simulink model "Supply_Chain_III"  (R2018b)
settings: Solver=VariableStepAuto  StartTime=0.0  StopTime=n_T  RelTol=1e-3
undefined symbols (not defined in the file or in its folder): m, MTBF_h, n, yoi
libraries: simulink x6
settings Model: Creator=Jorrit de Jong  LastModifiedBy=Jorrit de Jong

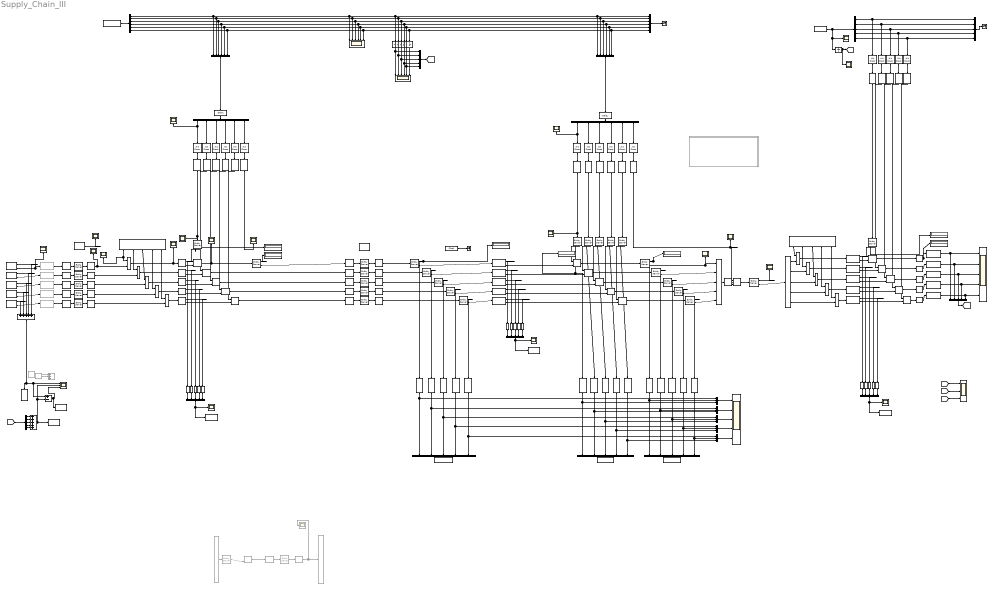
== system Supply_Chain_III ==
  note: KPI to indicate the in-time or delayed deliveries
  note: KPI to indicate the component availability on AI
  note: Performance measurement
  note: Local Warehouse
  note: Scopes
  note: KPI to indicate demanded terminal capacity
  note: Shedule Agent
  note: Control agent
  note: Terminal
  note: Island
  note: Performance measurement JIT
  note: Performance measurement
  note: Control agent
  note: Nr of parts departed
  note: Failure Agent
  note: Performance measurement
  note: KPI to measure the inventory level relative to the sigma level
  note: Source
  Add : Sum  Inputs=+++++
  Add1 : Sum  Inputs=+++++
  Add2 : Sum  Inputs=+-
  Add3 : Sum  Commented=on  Inputs=+++
  Arrived spares : Display
  Blade terminator : EntityTerminator  InputPortMessageModes=m  NumberEntitiesArrived=on
      settings: OutputPortMap=o0
  C terminator : EntityTerminator  InputPortMessageModes=m  NumberEntitiesArrived=on
      settings: OutputPortMap=o0
  Components arrived : Scope  NumInputPorts=5
  Constant : Constant  Commented=on  Value=5*20
  Constant1 : Constant  Commented=on  Value=5*20
  Counter : EntityServer  InputPortMessageModes=m  OutputPortMessageModes=n,m  Capacity=inf  ServiceTimeValue=0  NumberEntitiesDeparted=on
      settings: OutputPortMap=o0,o9
  Counter2 : EntityServer  InputPortMessageModes=m  OutputPortMessageModes=n,m  Capacity=inf  ServiceTimeValue=0  NumberEntitiesDeparted=on
      settings: OutputPortMap=o0,o9
  D terminator : EntityTerminator  InputPortMessageModes=m  NumberEntitiesArrived=on
      settings: OutputPortMap=o0
  DC transport signal : Scope
  DC trigger : Scope
  Data Type Conversion{,1..34} (35 alike) : DataTypeConversion
  Demand - delivery flow : Scope  NumInputPorts=3
  Demux : Demux  Outputs=6
  Demux1 : Demux  Outputs=5
  Demux2 : Demux  Outputs=5
  Demux3 : Demux  Outputs=6
  Demux5 : Demux  Outputs=6
  Departed/Arrived components : Scope  NumInputPorts=3
  Digital Clock : DigitalClock
  Display : Display
  Display1 : Display
  Display2 : Display
  E terminator : EntityTerminator  InputPortMessageModes=m  NumberEntitiesArrived=on
      settings: OutputPortMap=o0
  Entity Input Switch : EntityInputSwitch  Commented=on  InputPortMessageModes=m,m,m,m,m  OutputPortMessageModes=m  NumberInputPorts=5
      settings: InputPortMap=u1,u2,u3,u4,u5
  Entity Input Switch{1..5,7..11} (10 alike) : EntityInputSwitch  InputPortMessageModes=m,m  OutputPortMessageModes=m
  Entity Input Switch6 : EntityInputSwitch  InputPortMessageModes=m,m,m,m,m  OutputPortMessageModes=m  NumberInputPorts=5
      settings: InputPortMap=u1,u2,u3,u4,u5
  Entity Output Switch : EntityOutputSwitch  InputPortMessageModes=m  OutputPortMessageModes=m,m,m,m,m  NumberOutputPorts=5  SwitchingCriterion=From attribute  SwitchAttributeName=PartNumber
      settings: OutputPortMap=o0,o1,o2,o3,o4
  Entity Output Switch1 : EntityOutputSwitch  Commented=on  InputPortMessageModes=m  OutputPortMessageModes=m,m,m,m,m  NumberOutputPorts=5  SwitchingCriterion=From attribute  SwitchAttributeName=PartNumber
      settings: OutputPortMap=o0,o1,o2,o3,o4
  Entity Gate{,1..9,11..16} (16 alike) : EntityGate  InputPortMessageModes=m,m  OutputPortMessageModes=m  OperatingMode=Release gate
  Entity Gate10 : EntityGate  Commented=on  InputPortMessageModes=m,m  OutputPortMessageModes=m  OperatingMode=Release gate
  Entity Generator : EntityGenerator  OutputPortMessageModes=n,m  Period=MTBF_h(1,yoi)  AttributeName=PartNumber  NumberEntitiesDeparted=on  EntityType=Structured  EntityTypeName=Part
      settings: OutputPortMap=o0,o3
  Entity Generator1 : EntityGenerator  OutputPortMessageModes=n,m  Period=MTBF_h(2,yoi)  AttributeName=PartNumber  AttributeInitialValue=2  NumberEntitiesDeparted=on  EntityType=Structured  EntityTypeName=Part
      settings: OutputPortMap=o0,o3
  Entity Generator{5..16,18..22} (17 alike) : EntityGenerator  InputPortMessageModes=m  OutputPortMessageModes=m  GenerationMethod=Event-based  AttributeName=entity  AttributeInitialValue=0  EntityTypeName=Entity
      settings: InputPortMap=u0
  Entity Generator2 : EntityGenerator  OutputPortMessageModes=n,m  Period=MTBF_h(3,yoi)  AttributeName=PartNumber  AttributeInitialValue=3  NumberEntitiesDeparted=on  EntityType=Structured  EntityTypeName=Part
      settings: OutputPortMap=o0,o3
  Entity Generator3 : EntityGenerator  OutputPortMessageModes=n,m  Period=MTBF_h(4,yoi)  AttributeName=PartNumber  AttributeInitialValue=4  NumberEntitiesDeparted=on  EntityType=Structured  EntityTypeName=Part
      settings: OutputPortMap=o0,o3
  Entity Generator4 : EntityGenerator  OutputPortMessageModes=n,m  Period=MTBF_h(5,yoi)  AttributeName=PartNumber  AttributeInitialValue=5  NumberEntitiesDeparted=on  EntityType=Structured  EntityTypeName=Part
      settings: OutputPortMap=o0,o3
  Entity Queue{,1..9} (10 alike) : EntityQueue  InputPortMessageModes=m  OutputPortMessageModes=n,m  Capacity=20  NumberEntitiesInBlock=on
      settings: OutputPortMap=o1,o5
  Entity Queue{10..14} (5 alike) : EntityQueue  Commented=through  InputPortMessageModes=m  OutputPortMessageModes=m  Capacity=1
      settings: OutputPortMap=o5
  Entity Server{,1..3,9..20} (16 alike) : EntityServer  InputPortMessageModes=m  OutputPortMessageModes=n,m  Capacity=inf  ServiceTimeValue=0  NumberEntitiesDeparted=on
      settings: OutputPortMap=o0,o9
  Entity Server{4..8} (5 alike) : EntityServer  InputPortMessageModes=m  OutputPortMessageModes=m  Capacity=inf  ServiceTimeSource=MATLAB action  ServiceTimeValue=20  ServiceTimeAction=dt = normrnd(D(1,3),ts_sigma_distance(1,3));
  Entity Store{,1..4} (5 alike) : EntityStore  InputPortMessageModes=m  OutputPortMessageModes=n,m  Capacity=20  NumberEntitiesInBlock=on
      settings: OutputPortMap=o1,o4
  Entity Store6 : EntityStore  InputPortMessageModes=m  OutputPortMessageModes=m  Capacity=inf
      settings: OutputPortMap=o4
  Failures : Display
  Failures cumulated : Scope
  Failures3 : Display
  From Workspace : FromWorkspace  VariableName=Failure_events  SampleTime=0
  From Workspace1 : FromWorkspace  VariableName=Schedule_data  SampleTime=0
  Gearbox terminator : EntityTerminator  InputPortMessageModes=m  NumberEntitiesArrived=on
      settings: OutputPortMap=o0
  Hit Crossing{,1..16} (17 alike) : HitCross  OutputPortMessageModes=m  HitCrossingDirection=rising  HitCrossingOutputType=Message
  Ini supply creator : Subsystem
  Ini supply creator1 : Subsystem
  Integrator{,3..8} (7 alike) : Integrator
  Inventory level island : Scope
  Inventory level local warehouse : Scope
  Inventory level terminal : Scope
  JIT Scope : Scope  NumInputPorts=5
  Loading : EntityServer  Commented=on  InputPortMessageModes=m  OutputPortMessageModes=m  Capacity=inf  ServiceTimeValue=1
  Mux : Mux  Inputs=6
  Mux{1,4..9,15,17} (9 alike) : Mux  Inputs=5
  Mux10 : Mux  Inputs=6
  Mux{3,11..14} (5 alike) : Mux  Inputs=3
  Mux2 : Mux  Inputs=6
  Overall DC releaser : Scope
  Passed components : Display
  Post DC trigger : Scope
  Pre DC storage{,1..4} (5 alike) : Scope
  Resource Acquirer{,1..4} (5 alike) : EntityResourceAcquirer  InputPortMessageModes=m  OutputPortMessageModes=m  ResourceName=LD_trucks
      settings: OutputPortMap=o3
  Resource Acquirer{6..10} (5 alike) : EntityResourceAcquirer  InputPortMessageModes=m  OutputPortMessageModes=m
      settings: OutputPortMap=o3
  Resource Acquirer5 : EntityResourceAcquirer  Commented=on  InputPortMessageModes=m  OutputPortMessageModes=m
      settings: OutputPortMap=o3
  Resource Releaser{,1..4} (5 alike) : EntityResourceReleaser  InputPortMessageModes=m  OutputPortMessageModes=m  ResourceToRelease=Selected  ResourceName=LD_trucks
  Resource Releaser{6..10} (5 alike) : EntityResourceReleaser  InputPortMessageModes=m  OutputPortMessageModes=m
  Resource Releaser5 : EntityResourceReleaser  Commented=on  InputPortMessageModes=m  OutputPortMessageModes=m
  Resource Pool : EntityResourcePool  ResourceName=LD_trucks  ResourceAmount=30  AverageUtilization=on
      settings: OutputPortMap=o1
  Resource Pool1 : EntityResourcePool  ResourceAmount=n_R
  Road transport : EntityServer  Commented=on  InputPortMessageModes=m  OutputPortMessageModes=m  Capacity=inf  ServiceTimeSource=MATLAB action  ServiceTimeValue=20  ServiceTimeAction=dt = normrnd(D(3,4),ts_sigma_distance(3,4));
  Road transport troughput : Scope  Commented=on
  Road transport{1..5} (5 alike) : EntityServer  InputPortMessageModes=m  OutputPortMessageModes=m  Capacity=inf  ServiceTimeSource=MATLAB action  ServiceTimeValue=20  ServiceTimeAction=dt = normrnd(D(3,4),ts_sigma_distance(3,4));
  Schedule data : Scope  NumInputPorts=6
  Schedule data accumulated : Scope  NumInputPorts=6
  Scope4 : Scope
  Sea Transport : EntityServer  InputPortMessageModes=m  OutputPortMessageModes=n,m  Capacity=inf  ServiceTimeSource=MATLAB action  ServiceTimeValue=50  ServiceTimeAction=dt = normrnd(ts_vessel,2);  NumberEntitiesDeparted=on
      settings: OutputPortMap=o0,o9
  Sea transport post releaser : Scope
  Sea transport releaser : Scope
  Sea transport signal : Scope
  Sea transport sope : Scope
  Sea transport trigger : Scope
  Switched transport delay for linearization : TransportDelay  DelayTime=3  PadeOrder=1
  Switched transport delay for linearization1 : TransportDelay  PadeOrder=1
  Terminal trigger system : Subsystem  Commented=on
  Terminator1 : Terminator
  Terminator2 : Terminator
  Terminator4 : Terminator
  To Workspace : ToWorkspace  VariableName=inventory_level_island
      settings: Save2DSignal=2-D array (concatenate along first dimension)
  To Workspace1 : ToWorkspace  VariableName=com_caller
      settings: Save2DSignal=2-D array (concatenate along first dimension)
  To Workspace2 : ToWorkspace  VariableName=com_released
      settings: Save2DSignal=2-D array (concatenate along first dimension)
  To Workspace3 : ToWorkspace  VariableName=com_arrivals
      settings: Save2DSignal=2-D array (concatenate along first dimension)
  To Workspace4 : ToWorkspace  VariableName=inventory_level_terminal
      settings: Save2DSignal=2-D array (concatenate along first dimension)
  To Workspace5 : ToWorkspace  VariableName=inventory_level_LW
      settings: Save2DSignal=2-D array (concatenate along first dimension)
  To Workspace6 : ToWorkspace  VariableName=departed_comps
      settings: Save2DSignal=2-D array (concatenate along first dimension)
  To Workspace7 : ToWorkspace  VariableName=arrived_comps
      settings: Save2DSignal=2-D array (concatenate along first dimension)
  To Workspace8 : ToWorkspace  VariableName=n_comps_in_sc
      settings: Save2DSignal=2-D array (concatenate along first dimension)
  wires:
  Data Type Conversion15/1 -> Mux6/5  "Transformers"
  Entity Queue6/1 -> Data Type Conversion9/1
  Counter/1 -> Passed components/1
  Hit Crossing7/1 -> Entity Generator12/1
  Entity Queue2/2 -> Entity Gate2/2
  Entity Queue1/2 -> Entity Gate1/2
  Entity Gate1/1 -> Gearbox terminator/1
  Entity Gate/1 -> Blade terminator/1
  Hit Crossing1/1 -> Entity Generator6/1
  Demux/1 -> Schedule data/1, Integrator3/1, Mux2/1, Mux/1, Mux10/1  "A"
  Entity Output Switch/5 -> Entity Input Switch5/2
  Resource Releaser/1 -> Entity Input Switch7/2, Pre DC storage4/1
  Entity Generator2/1 -> Add/3
  Entity Input Switch3/1 -> Entity Queue2/1
  Constant/1 -> Add3/1
  Entity Store3/1 -> Data Type Conversion14/1
  Constant1/1 -> Add3/2
  Demux2/1 -> Add1/1
  Integrator3/1 -> Mux17/1, Schedule data accumulated/1
  Entity Server5/1 -> Resource Releaser1/1
  Demux2/2 -> Add1/2
  Entity Queue8/1 -> Data Type Conversion11/1
  Entity Server3/1 -> Display2/1, Data Type Conversion2/1
  Data Type Conversion32/1 -> Mux15/3, Components arrived/3
  Entity Server/1 -> Display/1, Data Type Conversion1/1
  Integrator4/1 -> Mux17/2, Schedule data accumulated/2
  Entity Gate7/1 -> Resource Acquirer8/1
  Entity Server11/2 -> Entity Queue8/1
  Hit Crossing4/1 -> Entity Generator9/1
  Data Type Conversion31/1 -> Mux15/2, Components arrived/2
  Data Type Conversion4/1 -> Mux4/2  "Gearboxes"
  Entity Generator14/1 -> Entity Gate8/1
  Demux2/3 -> Add1/3
  Entity Queue4/2 -> Entity Gate4/2
  Entity Generator3/1 -> Add/2
  Add/1 -> To Workspace6/1, Add2/1, Departed/Arrived components/1  "Departs"
  Integrator8/1 -> Schedule data accumulated/6
  Demux/2 -> Schedule data/2, Integrator4/1, Mux2/2, Mux/2, Mux10/2  "B"
  [Sche_comps] -> Demand - delivery flow/2  "Scheduled"
  Entity Generator1/1 -> Add/4
  Entity Server6/1 -> Resource Releaser2/1
  Resource Releaser1/1 -> Entity Input Switch8/2
  Entity Gate9/1 -> Resource Acquirer10/1
  Entity Queue3/1 -> Data Type Conversion6/1
  Data Type Conversion34/1 -> Mux15/5, Components arrived/5
  Demux3/3 -> Hit Crossing8/1
  Demux3/5 -> Hit Crossing10/1
  Entity Queue10/1 -> Resource Acquirer/1
  Resource Acquirer3/1 -> Entity Server7/1
  Mux11/1 -> JIT Scope/2  "Gearboxes"
  Entity Queue7/1 -> Data Type Conversion10/1
  Resource Acquirer1/1 -> Entity Server5/1
  Entity Queue11/1 -> Resource Acquirer1/1
  Entity Queue12/1 -> Resource Acquirer2/1
  Mux15/1 -> [Arr_comps]
  Entity Server1/1 -> Failures/1
  Data Type Conversion12/1 -> Mux5/5  "Transformers"
  Entity Server12/2 -> Entity Queue9/1
  Data Type Conversion16/1 -> Mux6/1  "Blades"
  Resource Acquirer2/1 -> Entity Server6/1
  Entity Queue8/2 -> Entity Gate14/2
  Data Type Conversion33/1 -> Mux15/4, Components arrived/4
  Entity Generator13/1 -> Entity Gate7/1
  Integrator7/1 -> Mux17/5, Schedule data accumulated/5
  Data Type Conversion3/1 -> Mux4/1  "Blades"
  Gearbox terminator/1 -> Data Type Conversion31/1
  Entity Gate3/1 -> D terminator/1
  Data Type Conversion30/1 -> Mux15/1, Components arrived/1
  Data Type Conversion5/1 -> Mux4/3  "Generators"
  Road transport1/1 -> Resource Releaser6/1
  Entity Queue3/2 -> Entity Gate3/2
  Entity Server15/1 -> Data Type Conversion24/1
  Integrator/1 -> Failures cumulated/1, [Fail_comps]
  Data Type Conversion7/1 -> Mux4/5  "Transformers"
  Entity Generator22/1 -> Entity Gate4/1
  Integrator5/1 -> Mux17/3, Schedule data accumulated/3
  D terminator/1 -> Data Type Conversion33/1
  Entity Generator19/1 -> Entity Gate1/1
  Data Type Conversion20/1 -> Mux13/1, Mux9/4  "Arrivals"
  Hit Crossing/1 -> Entity Generator5/1
  Demux/6 -> Schedule data/6, Integrator8/1, Mux2/6, Mux/6, Mux10/6  "t"
  From Workspace/1 -> Integrator/1, Scope4/1, Demux1/1
  Entity Gate2/1 -> C terminator/1
  Resource Releaser4/1 -> Entity Input Switch11/2
  Demux/3 -> Schedule data/3, Integrator5/1, Mux2/3, Mux/3, Mux10/3  "C"
  Demux2/4 -> Add1/4
  Hit Crossing14/1 -> Entity Generator20/1
  Demux3/6 -> Hit Crossing11/1
  Mux3/1 -> JIT Scope/1  "Blades"
  Resource Acquirer/1 -> Entity Server4/1
  E terminator/1 -> Data Type Conversion34/1
  Resource Releaser2/1 -> Entity Input Switch9/2
  Entity Generator21/1 -> Entity Gate3/1
  Demux5/1 -> Hit Crossing/1, Sea transport signal/1
  Mux/1 -> Terminator4/1
  Demux/4 -> Schedule data/4, Integrator6/1, Mux2/4, Mux/4, Mux10/4  "D"
  Resource Releaser3/1 -> Entity Input Switch10/2
  Digital Clock/1 -> Terminator1/1
  Counter/2 -> Resource Acquirer6/1
  Data Type Conversion11/1 -> Mux5/4  "Rotorhubs"
  Ini supply creator1/3(C) -> Entity Input Switch9/1
  Mux2/1 -> Switched transport delay for linearization/1
  Entity Generator15/1 -> Entity Gate9/1
  Entity Queue9/1 -> Data Type Conversion12/1
  Entity Gate5/1 -> Post DC trigger/1, Counter/1
  Entity Generator10/1 -> Entity Gate16/1, Sea transport releaser/1
  Mux10/1 -> Switched transport delay for linearization1/1
  Hit Crossing16/1 -> Entity Generator22/1
  From Workspace1/1 -> Demux/1
  Entity Generator16/1 -> Overall DC releaser/1
  Hit Crossing15/1 -> Entity Generator21/1
  Demux3/2 -> Hit Crossing7/1
  Demux1/2 -> Mux1/2, Hit Crossing13/1  "B"
  Hit Crossing10/1 -> Entity Generator15/1
  Demux1/1 -> Mux1/1, Hit Crossing12/1  "A"
  Mux5/1 -> To Workspace4/1, Inventory level terminal/1
  Mux17/1 -> [Sche_comps]
  Entity Generator11/1 -> DC trigger/1, Counter2/1
  Entity Output Switch/3 -> Entity Input Switch3/2
  Entity Input Switch11/1 -> Entity Store4/1
  Entity Generator4/2 -> Entity Queue14/1
  Data Type Conversion8/1 -> Mux5/1  "Blades"
  Mux9/1 -> To Workspace3/1
  Entity Generator7/1 -> Entity Server18/1
  Entity Output Switch/2 -> Entity Input Switch2/2
  Demux1/4 -> Mux1/4, Hit Crossing15/1  "D"
  Entity Generator8/1 -> Entity Server19/1
  Entity Generator5/1 -> Sea transport trigger/1, Entity Server2/1
  Blade terminator/1 -> Arrived spares/1, Data Type Conversion30/1
  Hit Crossing9/1 -> Entity Generator14/1
  Demux1/5 -> Mux1/5, Hit Crossing16/1  "E"
  Data Type Conversion23/1 -> Mux8/3, Mux12/2  "Released"
  Switched transport delay for linearization1/1 -> Demux3/1
  Entity Server10/2 -> Entity Queue7/1
  Switched transport delay for linearization/1 -> Demux5/1
  Data Type Conversion21/1 -> Mux9/5, Mux14/1  "Arrivals"
  Hit Crossing12/1 -> Entity Generator18/1
  [Fail_comps] -> Demand - delivery flow/1  "Failures"
  Add2/1 -> To Workspace8/1, Departed/Arrived components/3  "Result"
  Entity Server/2 -> Entity Input Switch6/1, Sea transport post releaser/1
  Demux1/3 -> Mux1/3, Hit Crossing14/1  "C"
  C terminator/1 -> Data Type Conversion32/1
  Data Type Conversion10/1 -> Mux5/3  "Generators"
  Demux3/1 -> Hit Crossing6/1, DC transport signal/1
  Entity Store/2 -> Entity Gate5/2
  Entity Queue14/1 -> Resource Acquirer4/1
  Data Type Conversion1/1 -> Mux3/2, Mux8/1  "Released"
  Entity Server1/2 -> Entity Gate/1
  Mux12/1 -> JIT Scope/3  "Generators"
  Data Type Conversion18/1 -> Mux11/1, Mux9/2  "Arrivals"
  Entity Server14/1 -> Data Type Conversion23/1
  Entity Queue4/1 -> Data Type Conversion7/1
  Entity Generator/2 -> Pre DC storage2/1, Entity Queue10/1
  Entity Store4/1 -> Data Type Conversion15/1
  Entity Gate4/1 -> E terminator/1
  Hit Crossing8/1 -> Entity Generator13/1
  Entity Server4/1 -> Resource Releaser/1
  Demux5/5 -> Hit Crossing4/1
  Entity Server13/1 -> Data Type Conversion22/1
  Data Type Conversion25/1 -> Mux8/5, Mux14/2  "Released"
  Entity Generator1/2 -> Entity Queue11/1
  Entity Queue5/1 -> Data Type Conversion8/1
  Mux6/1 -> To Workspace5/1, Inventory level local warehouse/1
  Data Type Conversion22/1 -> Mux11/2, Mux8/2  "Released"
  Mux14/1 -> JIT Scope/5  "Transformer"
  Entity Queue9/2 -> Entity Gate15/2
  Entity Input Switch5/1 -> Entity Queue4/1
  Entity Queue6/2 -> Entity Gate12/2
  Entity Generator4/1 -> Add/1
  Data Type Conversion2/1 -> Mux3/1, Mux9/1  "Arrivals"
  Mux8/1 -> To Workspace2/1
  Hit Crossing13/1 -> Entity Generator19/1
  Data Type Conversion29/1 -> Mux7/5, Mux14/3  "Caller"
  Entity Server17/1 -> Data Type Conversion26/1
  Demux5/4 -> Hit Crossing3/1
  Entity Generator12/1 -> Entity Gate6/1
  Entity Server7/1 -> Resource Releaser3/1
  Entity Server18/1 -> Data Type Conversion27/1
  Entity Generator20/1 -> Entity Gate2/1
  Mux7/1 -> To Workspace1/1
  Entity Server20/1 -> Data Type Conversion29/1
  Data Type Conversion28/1 -> Mux13/3, Mux7/4  "Caller"
  Entity Server19/1 -> Data Type Conversion28/1
  Demux2/5 -> Add1/5
  Resource Releaser8/1 -> Entity Server10/1
  Data Type Conversion14/1 -> Mux6/4  "Rotorhubs"
  Entity Queue13/1 -> Resource Acquirer3/1
  Mux13/1 -> JIT Scope/4  "Rotor hubs"
  Entity Input Switch8/1 -> Entity Store1/1
  Entity Queue2/1 -> Data Type Conversion5/1
  Entity Server19/2 -> Entity Gate14/1
  Entity Server15/2 -> Entity Input Switch6/4
  Entity Server17/2 -> Entity Gate12/1
  Hit Crossing3/1 -> Entity Generator8/1
  Data Type Conversion19/1 -> Mux12/1, Mux9/3  "Arrivals"
  Entity Server16/1 -> Data Type Conversion25/1
  Data Type Conversion24/1 -> Mux13/2, Mux8/4  "Released"
  Hit Crossing2/1 -> Entity Generator7/1
  Data Type Conversion27/1 -> Mux12/3, Mux7/3  "Caller"
  Entity Generator/1 -> Add/5
  Entity Server10/1 -> Data Type Conversion19/1
  Entity Server13/2 -> Entity Input Switch6/2
  Data Type Conversion9/1 -> Mux5/2  "Gearboxes"
  Data Type Conversion6/1 -> Mux4/4  "Rotorhubs"
  Resource Releaser10/1 -> Entity Server12/1
  Entity Server20/2 -> Entity Gate15/1
  Entity Gate12/1 -> Entity Server13/1
  Ini supply creator1/2(B) -> Entity Input Switch8/1
  Entity Generator3/2 -> Entity Queue13/1
  Resource Releaser9/1 -> Entity Server11/1
  Entity Server9/1 -> Data Type Conversion18/1
  Entity Input Switch2/1 -> Entity Queue1/1
  Ini supply creator/3(C) -> Entity Input Switch3/1
  Demux5/6 -> Hit Crossing5/1
  Hit Crossing5/1 -> Entity Generator10/1
  Demux5/3 -> Hit Crossing2/1
  Entity Server3/2 -> Entity Queue5/1
  Mux4/1 -> To Workspace/1, Inventory level island/1
  Integrator6/1 -> Mux17/4, Schedule data accumulated/4
  Entity Store2/2 -> Entity Gate7/2
  Add1/1 -> To Workspace7/1, Departed/Arrived components/2, Add2/2  "Arrivals"
  Demux5/2 -> Hit Crossing1/1
  Entity Store4/2 -> Entity Gate9/2
  Entity Store3/2 -> Entity Gate8/2
  Entity Store1/2 -> Entity Gate6/2
  Entity Queue7/2 -> Entity Gate13/2
  Ini supply creator/2(B) -> Entity Input Switch2/1
  Demux3/4 -> Hit Crossing9/1
  Entity Gate13/1 -> Entity Server14/1
  Ini supply creator/5(E) -> Entity Input Switch5/1
  Hit Crossing6/1 -> Entity Generator11/1
  Entity Gate11/1 -> Entity Server/1
  Ini supply creator1/5(E) -> Entity Input Switch11/1
  Entity Server12/1 -> Data Type Conversion21/1
  Entity Generator9/1 -> Entity Server20/1
  Entity Input Switch7/1 -> Pre DC storage/1, Entity Store/1
  Entity Server9/2 -> Entity Queue6/1
  Resource Acquirer4/1 -> Entity Server8/1
  Entity Queue1/1 -> Data Type Conversion4/1
  [Arr_comps] -> Demux2/1  "Delivered"
  Entity Output Switch/1 -> Entity Input Switch1/2
  Resource Releaser7/1 -> Entity Server9/1
  Entity Queue/1 -> Data Type Conversion3/1
  Data Type Conversion13/1 -> Mux6/3  "Generators"
  Demux/5 -> Schedule data/5, Integrator7/1, Mux2/5, Mux/5, Mux10/5  "E"
  Ini supply creator/1(A) -> Entity Input Switch1/1
  Entity Store2/1 -> Data Type Conversion13/1
  Counter2/1 -> Failures3/1
  Entity Store1/1 -> Data Type Conversion17/1
  Data Type Conversion17/1 -> Mux6/2  "Gearboxes"
  Entity Store/1 -> Data Type Conversion16/1
  Data Type Conversion/1 -> Mux3/3, Mux7/1  "Caller"
  Counter2/2 -> Entity Gate5/1
  Ini supply creator/4(D) -> Entity Input Switch4/1
  Entity Generator6/1 -> Entity Server17/1
  Hit Crossing11/1 -> Entity Generator16/1
  Entity Queue5/2 -> Entity Gate11/2
  [Arr_comps] -> Demand - delivery flow/3  "Delivered"
  Ini supply creator1/1(A) -> Pre DC storage1/1, Entity Input Switch7/1
  Entity Gate14/1 -> Entity Server15/1
  Entity Server16/2 -> Entity Input Switch6/5
  Entity Output Switch/4 -> Entity Input Switch4/2
  Entity Server18/2 -> Entity Gate13/1
  Ini supply creator1/4(D) -> Entity Input Switch10/1
  Mux1/1 -> Terminator2/1
  Entity Gate6/1 -> Resource Acquirer7/1
  Entity Gate15/1 -> Entity Server16/1
  Entity Input Switch10/1 -> Entity Store3/1
  Entity Server2/2 -> Entity Gate11/1
  Entity Input Switch1/1 -> Entity Queue/1
  Entity Generator18/1 -> Entity Server1/1
  Entity Input Switch4/1 -> Entity Queue3/1
  Entity Server2/1 -> Display1/1, Data Type Conversion/1
  Entity Queue/2 -> Entity Gate/2
  Entity Server14/2 -> Entity Input Switch6/3
  Entity Input Switch9/1 -> Entity Store2/1
  Entity Server11/1 -> Data Type Conversion20/1
  Entity Server8/1 -> Resource Releaser4/1
  Entity Generator2/2 -> Entity Queue12/1
  Data Type Conversion26/1 -> Mux11/3, Mux7/2  "Caller"
  Resource Pool/1 -> Pre DC storage3/1
  Entity Store6/1 -> Entity Gate16/2
  Entity Gate16/1 -> Sea Transport/1
  Entity Input Switch6/1 -> Entity Store6/1
  Sea Transport/1 -> Sea transport sope/1
  Sea Transport/2 -> Entity Output Switch/1
  Loading/1 -> Entity Gate10/2
  Entity Input Switch/1 -> Loading/1
  Road transport/1 -> Resource Releaser5/1
  Entity Gate10/1 -> Resource Acquirer5/1
  Resource Acquirer5/1 -> Road transport/1
  Resource Releaser5/1 -> Entity Output Switch1/1, Road transport troughput/1
  Resource Releaser6/1 -> Entity Server3/1
  Resource Acquirer6/1 -> Road transport1/1
  Resource Acquirer7/1 -> Road transport2/1
  Road transport2/1 -> Resource Releaser7/1
  Resource Acquirer8/1 -> Road transport3/1
  Road transport3/1 -> Resource Releaser8/1
  Resource Acquirer9/1 -> Road transport4/1
  Road transport4/1 -> Resource Releaser9/1
  Resource Acquirer10/1 -> Road transport5/1
  Road transport5/1 -> Resource Releaser10/1
  Entity Gate8/1 -> Resource Acquirer9/1

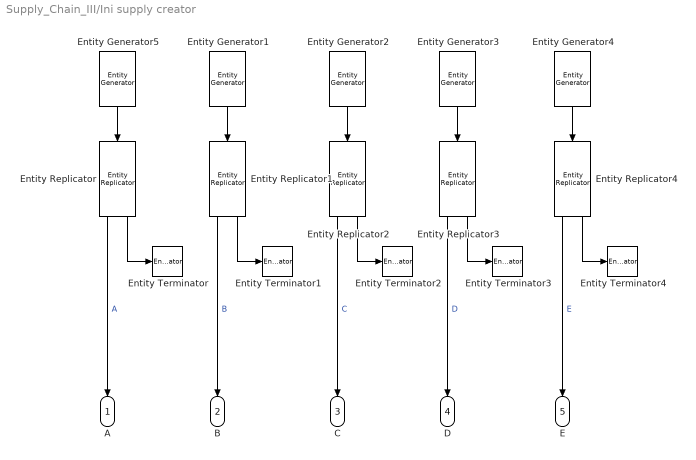
== system Supply_Chain_III/Ini supply creator ==
  Entity Generator1 : EntityGenerator  OutputPortMessageModes=m  Period=inf  AttributeName=PartNumber  AttributeInitialValue=2  EntityType=Structured  EntityTypeName=Part
  Entity Generator2 : EntityGenerator  OutputPortMessageModes=m  Period=inf  AttributeName=PartNumber  AttributeInitialValue=3  EntityType=Structured  EntityTypeName=Part
  Entity Generator3 : EntityGenerator  OutputPortMessageModes=m  Period=inf  AttributeName=PartNumber  AttributeInitialValue=4  EntityType=Structured  EntityTypeName=Part
  Entity Generator4 : EntityGenerator  OutputPortMessageModes=m  Period=inf  AttributeName=PartNumber  AttributeInitialValue=5  EntityType=Structured  EntityTypeName=Part
  Entity Generator5 : EntityGenerator  OutputPortMessageModes=m  Period=inf  AttributeName=PartNumber  EntityType=Structured  EntityTypeName=Part
  Entity Replicator{,1..4} (5 alike) : EntityReplicator  InputPortMessageModes=m  OutputPortMessageModes=m,m  ReplicasDepartFrom=Single output port  NumberReplicas=20
  Entity Terminator{,1..4} (5 alike) : EntityTerminator  InputPortMessageModes=m
  A : Outport
  B : Outport  Port=2
  C : Outport  Port=3
  D : Outport  Port=4
  E : Outport  Port=5
  wires:
  Entity Generator5/1 -> Entity Replicator/1
  Entity Replicator/2 -> Entity Terminator/1
  Entity Replicator/1 -> A/1  "A"
  Entity Replicator1/1 -> B/1  "B"
  Entity Generator1/1 -> Entity Replicator1/1
  Entity Replicator1/2 -> Entity Terminator1/1
  Entity Replicator2/1 -> C/1  "C"
  Entity Generator2/1 -> Entity Replicator2/1
  Entity Replicator2/2 -> Entity Terminator2/1
  Entity Replicator3/1 -> D/1  "D"
  Entity Generator3/1 -> Entity Replicator3/1
  Entity Replicator3/2 -> Entity Terminator3/1
  Entity Replicator4/1 -> E/1  "E"
  Entity Generator4/1 -> Entity Replicator4/1
  Entity Replicator4/2 -> Entity Terminator4/1

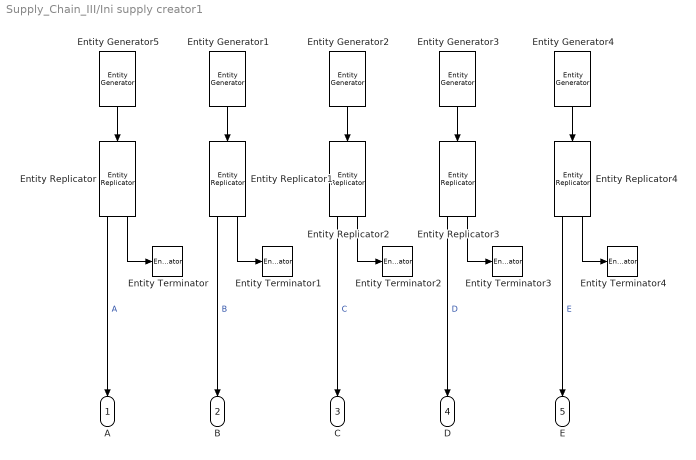
== system Supply_Chain_III/Ini supply creator1 ==
  Entity Generator1 : EntityGenerator  OutputPortMessageModes=m  Period=inf  AttributeName=PartNumber  AttributeInitialValue=2  EntityType=Structured  EntityTypeName=Part
  Entity Generator2 : EntityGenerator  OutputPortMessageModes=m  Period=inf  AttributeName=PartNumber  AttributeInitialValue=3  EntityType=Structured  EntityTypeName=Part
  Entity Generator3 : EntityGenerator  OutputPortMessageModes=m  Period=inf  AttributeName=PartNumber  AttributeInitialValue=4  EntityType=Structured  EntityTypeName=Part
  Entity Generator4 : EntityGenerator  OutputPortMessageModes=m  Period=inf  AttributeName=PartNumber  AttributeInitialValue=5  EntityType=Structured  EntityTypeName=Part
  Entity Generator5 : EntityGenerator  OutputPortMessageModes=m  Period=inf  AttributeName=PartNumber  EntityType=Structured  EntityTypeName=Part
  Entity Replicator{,1..4} (5 alike) : EntityReplicator  InputPortMessageModes=m  OutputPortMessageModes=m,m  ReplicasDepartFrom=Single output port  NumberReplicas=20
  Entity Terminator{,1..4} (5 alike) : EntityTerminator  InputPortMessageModes=m
  A : Outport
  B : Outport  Port=2
  C : Outport  Port=3
  D : Outport  Port=4
  E : Outport  Port=5
  wires:
  Entity Generator5/1 -> Entity Replicator/1
  Entity Replicator/2 -> Entity Terminator/1
  Entity Replicator/1 -> A/1  "A"
  Entity Replicator1/1 -> B/1  "B"
  Entity Generator1/1 -> Entity Replicator1/1
  Entity Replicator1/2 -> Entity Terminator1/1
  Entity Replicator2/1 -> C/1  "C"
  Entity Generator2/1 -> Entity Replicator2/1
  Entity Replicator2/2 -> Entity Terminator2/1
  Entity Replicator3/1 -> D/1  "D"
  Entity Generator3/1 -> Entity Replicator3/1
  Entity Replicator3/2 -> Entity Terminator3/1
  Entity Replicator4/1 -> E/1  "E"
  Entity Generator4/1 -> Entity Replicator4/1
  Entity Replicator4/2 -> Entity Terminator4/1

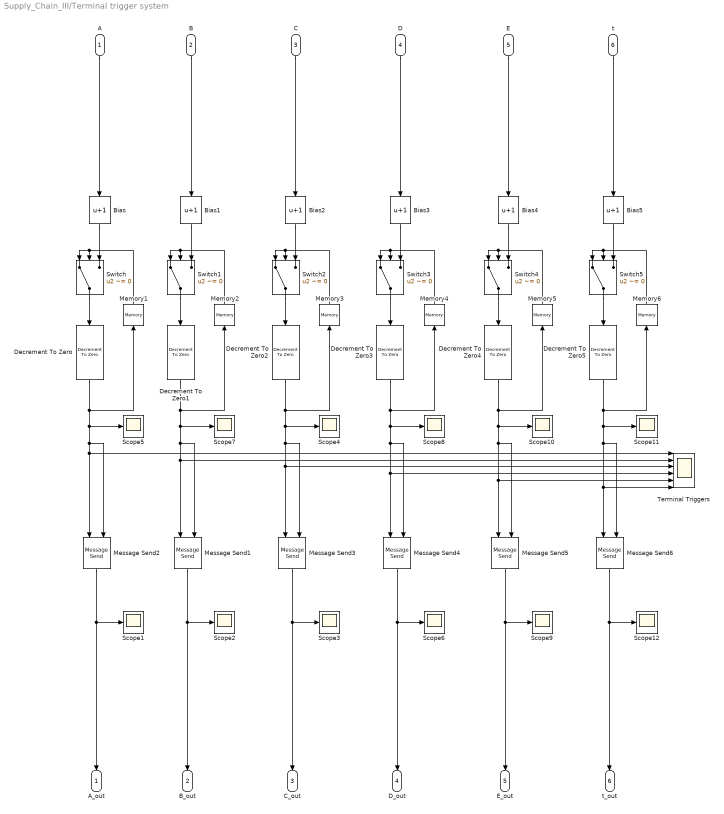
== system Supply_Chain_III/Terminal trigger system ==
  A : Inport
  B : Inport  Port=2
  C : Inport  Port=3
  D : Inport  Port=4
  E : Inport  Port=5
  t : Inport  Port=6
  Bias{,1..5} (6 alike) : Bias  Bias=1
  Decrement To Zero{,1..5} (6 alike) : simulink/Additional Math & Discrete/Additional Math: Increment - Decrement/Decrement To Zero
      settings: SourceProductName=Simulink  SourceProductBaseCode=SL
  Memory{1..6} (6 alike) : Memory
  Message Send{1..6} (6 alike) : MessageSend  OutputPortMessageModes=m  ShowEnablePort=on
      settings: InputPortMap=e0,u1
  Scope{1..12} (12 alike) : Scope
  Switch{,1..5} (6 alike) : Switch  Criteria=u2 ~= 0
  Terminal Triggers : Scope  NumInputPorts=6
  A_out : Outport
  B_out : Outport  Port=2
  C_out : Outport  Port=3
  D_out : Outport  Port=4
  E_out : Outport  Port=5
  t_out : Outport  Port=6
  wires:
  Bias1/1 -> Switch1/3
  Decrement To Zero/1 -> Message Send2/1, Terminal Triggers/1, Message Send2/2, Scope5/1, Memory1/1
  Switch/1 -> Decrement To Zero/1
  Decrement To Zero1/1 -> Message Send1/1, Terminal Triggers/2, Message Send1/2, Scope7/1, Memory2/1
  Memory1/1 -> Switch/2, Switch/1
  Memory2/1 -> Switch1/2, Switch1/1
  Bias/1 -> Switch/3
  Message Send1/1 -> Scope2/1, B_out/1
  Switch1/1 -> Decrement To Zero1/1
  Message Send2/1 -> Scope1/1, A_out/1
  A/1 -> Bias/1
  B/1 -> Bias1/1
  Bias2/1 -> Switch2/3
  Message Send3/1 -> Scope3/1, C_out/1
  Memory3/1 -> Switch2/2, Switch2/1
  Switch2/1 -> Decrement To Zero2/1
  C/1 -> Bias2/1
  Decrement To Zero2/1 -> Message Send3/1, Terminal Triggers/3, Message Send3/2, Scope4/1, Memory3/1
  Bias3/1 -> Switch3/3
  Message Send4/1 -> Scope6/1, D_out/1
  Memory4/1 -> Switch3/2, Switch3/1
  Switch3/1 -> Decrement To Zero3/1
  D/1 -> Bias3/1
  Decrement To Zero3/1 -> Message Send4/1, Terminal Triggers/4, Message Send4/2, Scope8/1, Memory4/1
  Bias4/1 -> Switch4/3
  Message Send5/1 -> Scope9/1, E_out/1
  Memory5/1 -> Switch4/2, Switch4/1
  Switch4/1 -> Decrement To Zero4/1
  E/1 -> Bias4/1
  Decrement To Zero4/1 -> Message Send5/1, Terminal Triggers/5, Message Send5/2, Scope10/1, Memory5/1
  Bias5/1 -> Switch5/3
  Message Send6/1 -> Scope12/1, t_out/1
  Decrement To Zero5/1 -> Terminal Triggers/6, Message Send6/1, Message Send6/2, Scope11/1, Memory6/1
  Switch5/1 -> Decrement To Zero5/1
  Memory6/1 -> Switch5/2, Switch5/1
  t/1 -> Bias5/1
